simulink model "PID_miniHopper_4_Pitch_Roll_Yaw_Contour_4"  (R2022b)
settings: Solver=VariableStepAuto  StartTime=0.0  StopTime=10  RelTol=1e-3
values from neighbouring files (symbols this model uses):
  hopper_ode = struct()    [MiniHopperParameters.m]
undefined symbols (not defined in the file or in its folder): A_rpy, B_rpy, Gain_pitch_U, Gain_roll_U, Gain_yaw_U, kT, VxLoop, VyLoop, XIC_rpy, XLoop, YLoop
libraries: simulink_extras x16, slpidlib x10
(part 1 of 2)
settings Model: Creator=User  LastModifiedBy=User

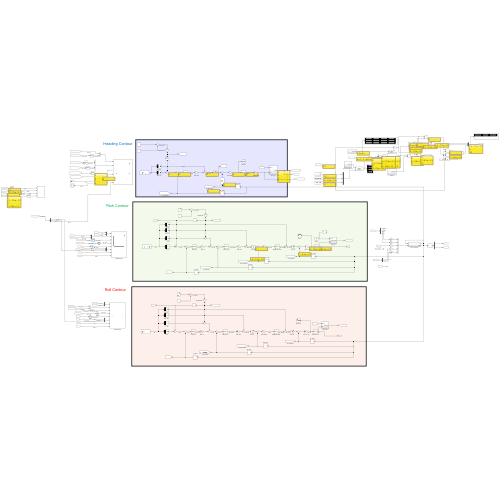
[thumbnail: Simulink's stored preview of the top-level diagram]
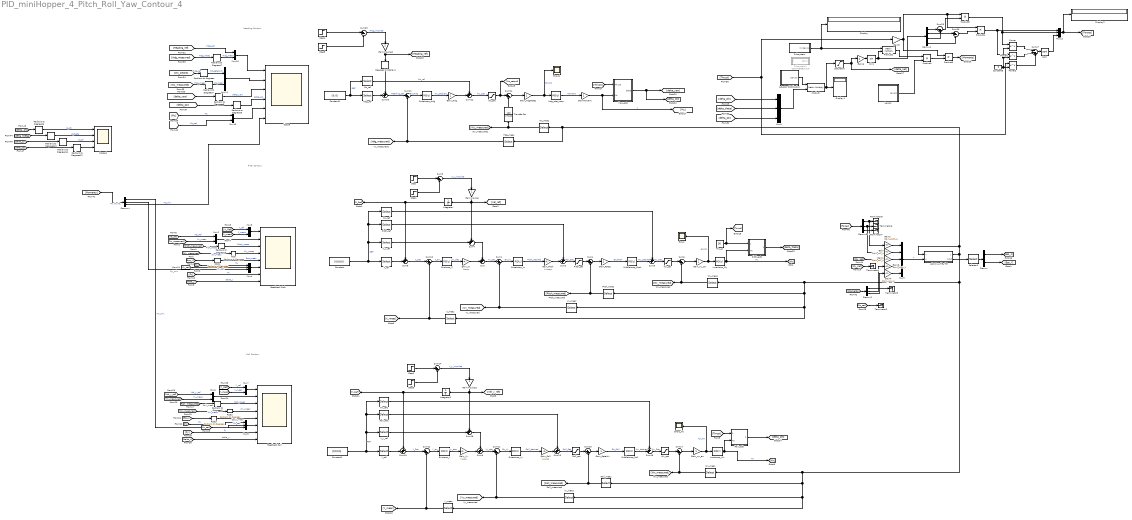
== system PID_miniHopper_4_Pitch_Roll_Yaw_Contour_4 ==
  note: Pitch Contour
  note: Roll Contour
  note: Heading Contour
  Actuator Distribution : Subsystem
  Constant : Constant  Value=[0;0;0;0]
  Constant1 : Constant  Value=[0;0;0;0]
  Constant2 : Constant  Value=[0; 0]
  Constant5 : Constant  Value=2
  Degrees to Radians : simulink_extras/Transformations/Degrees to Radians
  Demux : Demux  Outputs=2
  Demux1 : Demux
  Demux2 : Demux  Outputs=3
  Demux3 : Demux  Outputs=3
  Demux4 : Demux  Outputs=3
  Display : Display
  Display1 : Display
  Display2 : Display
  Errors : Scope
  Errors1 : Scope
  Errors_Wx : Scope
  ExoLoop_Y : slpidlib/PID Controller  Controller=PID  Form=Parallel  TimeDomain=Discrete-time  UseExternalTs=off  SampleTime=0.01  IntegratorMethod=Forward Euler  FilterMethod=Forward Euler  ControllerParametersSource=internal  P=0.1  I=0  UseKiTs=off  D=0  N=100  UseFilter=on  TunerSelectOption=Transfer Function Based (PID Tuner App)  InitialConditionSource=internal  InitialConditionForIntegrator=0  InitialConditionForFilter=0  DifferentiatorICPrevScaledInput=0  ExternalReset=none  TrackingMode=off  Kt=1  LimitOutput=off  SatLimitsSource=internal  UpperSaturationLimit=inf  LowerSaturationLimit=-inf  LinearizeAsGain=on  AntiWindupMode=none  Kb=1  LimitIntegrator=off  UpperIntegratorSaturationLimit=inf  LowerIntegratorSaturationLimit=-inf  POutMin=[]  POutMax=[]  IOutMin=[]  IOutMax=[]  DOutMin=[]  DOutMax=[]  NOutMin=[]  NOutMax=[]  SumOutMin=[]  SumOutMax=[]  SaturationOutMin=[]  SaturationOutMax=[]  PParamMin=[]  PParamMax=[]  IParamMin=[]  IParamMax=[]  DParamMin=[]  DParamMax=[]  NParamMin=[]  NParamMax=[]  KbParamMin=[]  KbParamMax=[]  KtParamMin=[]  KtParamMax=[]  KbOutMin=[]  KbOutMax=[]  KtOutMin=[]  KtOutMax=[]  IntegratorOutMin=[]  IntegratorOutMax=[]  FilterOutMin=[]  FilterOutMax=[]  SumI1OutMin=[]  SumI1OutMax=[]  SumI2OutMin=[]  SumI2OutMax=[]  SumI3OutMin=[]  SumI3OutMax=[]  SumI4OutMin=[]  SumI4OutMax=[]  SumDOutMin=[]  SumDOutMax=[]  DifferentiatorOutMin=[]  DifferentiatorOutMax=[]  FilterDiffOutCoefMin=[]  FilterDiffOutCoefMax=[]  ReciprocalOutMin=[]  ReciprocalOutMax=[]  SumDenOutMin=[]  SumDenOutMax=[]  SumNumOutMin=[]  SumNumOutMax=[]  DivideOutMin=[]  DivideOutMax=[]  UdiffTsProdOutMin=[]  UdiffTsProdOutMax=[]  NTsProdOutMin=[]  NTsProdOutMax=[]  UintegralTsProdOutMin=[]  UintegralTsProdOutMax=[]  UngainTsProdOutMin=[]  UngainTsProdOutMax=[]  ClampingZeroOutDataTypeStr=Inherit: Inherit via back propagation  ClampingZeroOutMin=[]  ClampingZeroOutMax=[]  FilterDenConstantOutDataTypeStr=Inherit: Inherit via back propagation  FilterDenConstantOutMin=[]  FilterDenConstantOutMax=[]  PCopyOutDataTypeStr=Inherit: Inherit via back propagation  PCopyOutMin=[]  PCopyOutMax=[]  NCopyOutDataTypeStr=Inherit: Inherit via back propagation  NCopyOutMin=[]  NCopyOutMax=[]  IntegratorContinuousStateAttributes=''  IntegratorStateMustResolveToSignalObject=off  IntegratorRTWStateStorageClass=Auto  FilterContinuousStateAttributes=''  FilterStateMustResolveToSignalObject=off  FilterRTWStateStorageClass=Auto  ParallelPVariant=InternalParameters  IdealPVariant=Disabled  IVariant=InternalParameters  DVariant=InternalParameters  IntegratorVariant=Discrete  SatVariant=Disabled  AWVariant=Passthrough  PCopyVariant=Disabled  TRVariant=Disabled  FdbkBlocksVariant=Forward  IdealPFdbkVariant=Disabled  SatFdbkVariant=Disabled  DerivativeFilterVariant=ForwardEulerFilter  NVariant=InternalParameters  NCopyVariant=Disabled  FilterICVariant=InternalICsFilter  IntegratorICVariant=InternalICs  ExternalResetVariant=Disabled  TRSumVariant=Passthrough  SumFdbkVariant=Disabled  SumVariant=Sum_PID  TsampFilterVariant=InternalTs  TsampNgainVariant=Passthrough  TsampIntegralVariant=Passthrough  ExternalSaturationOutDataTypeStr=Inherit: Same as second input
  ExoLoop_Z : slpidlib/PID Controller  Controller=PID  Form=Parallel  TimeDomain=Discrete-time  UseExternalTs=off  SampleTime=0.01  IntegratorMethod=Forward Euler  FilterMethod=Forward Euler  ControllerParametersSource=internal  P=0.1  I=0  UseKiTs=off  D=0  N=100  UseFilter=on  TunerSelectOption=Transfer Function Based (PID Tuner App)  InitialConditionSource=internal  InitialConditionForIntegrator=0  InitialConditionForFilter=0  DifferentiatorICPrevScaledInput=0  ExternalReset=none  TrackingMode=off  Kt=1  LimitOutput=off  SatLimitsSource=internal  UpperSaturationLimit=inf  LowerSaturationLimit=-inf  LinearizeAsGain=on  AntiWindupMode=none  Kb=1  LimitIntegrator=off  UpperIntegratorSaturationLimit=inf  LowerIntegratorSaturationLimit=-inf  POutMin=[]  POutMax=[]  IOutMin=[]  IOutMax=[]  DOutMin=[]  DOutMax=[]  NOutMin=[]  NOutMax=[]  SumOutMin=[]  SumOutMax=[]  SaturationOutMin=[]  SaturationOutMax=[]  PParamMin=[]  PParamMax=[]  IParamMin=[]  IParamMax=[]  DParamMin=[]  DParamMax=[]  NParamMin=[]  NParamMax=[]  KbParamMin=[]  KbParamMax=[]  KtParamMin=[]  KtParamMax=[]  KbOutMin=[]  KbOutMax=[]  KtOutMin=[]  KtOutMax=[]  IntegratorOutMin=[]  IntegratorOutMax=[]  FilterOutMin=[]  FilterOutMax=[]  SumI1OutMin=[]  SumI1OutMax=[]  SumI2OutMin=[]  SumI2OutMax=[]  SumI3OutMin=[]  SumI3OutMax=[]  SumI4OutMin=[]  SumI4OutMax=[]  SumDOutMin=[]  SumDOutMax=[]  DifferentiatorOutMin=[]  DifferentiatorOutMax=[]  FilterDiffOutCoefMin=[]  FilterDiffOutCoefMax=[]  ReciprocalOutMin=[]  ReciprocalOutMax=[]  SumDenOutMin=[]  SumDenOutMax=[]  SumNumOutMin=[]  SumNumOutMax=[]  DivideOutMin=[]  DivideOutMax=[]  UdiffTsProdOutMin=[]  UdiffTsProdOutMax=[]  NTsProdOutMin=[]  NTsProdOutMax=[]  UintegralTsProdOutMin=[]  UintegralTsProdOutMax=[]  UngainTsProdOutMin=[]  UngainTsProdOutMax=[]  ClampingZeroOutDataTypeStr=Inherit: Inherit via back propagation  ClampingZeroOutMin=[]  ClampingZeroOutMax=[]  FilterDenConstantOutDataTypeStr=Inherit: Inherit via back propagation  FilterDenConstantOutMin=[]  FilterDenConstantOutMax=[]  PCopyOutDataTypeStr=Inherit: Inherit via back propagation  PCopyOutMin=[]  PCopyOutMax=[]  NCopyOutDataTypeStr=Inherit: Inherit via back propagation  NCopyOutMin=[]  NCopyOutMax=[]  IntegratorContinuousStateAttributes=''  IntegratorStateMustResolveToSignalObject=off  IntegratorRTWStateStorageClass=Auto  FilterContinuousStateAttributes=''  FilterStateMustResolveToSignalObject=off  FilterRTWStateStorageClass=Auto  ParallelPVariant=InternalParameters  IdealPVariant=Disabled  IVariant=InternalParameters  DVariant=InternalParameters  IntegratorVariant=Discrete  SatVariant=Disabled  AWVariant=Passthrough  PCopyVariant=Disabled  TRVariant=Disabled  FdbkBlocksVariant=Forward  IdealPFdbkVariant=Disabled  SatFdbkVariant=Disabled  DerivativeFilterVariant=ForwardEulerFilter  NVariant=InternalParameters  NCopyVariant=Disabled  FilterICVariant=InternalICsFilter  IntegratorICVariant=InternalICs  ExternalResetVariant=Disabled  TRSumVariant=Passthrough  SumFdbkVariant=Disabled  SumVariant=Sum_PID  TsampFilterVariant=InternalTs  TsampNgainVariant=Passthrough  TsampIntegralVariant=Passthrough  ExternalSaturationOutDataTypeStr=Inherit: Same as second input
  Feedback Pitch : Scope  NumInputPorts=8
  Feedback Roll : Scope  NumInputPorts=8
  Gain : Gain  Gain=Gain_roll_U
  Gain1 : Gain  Gain=Gain_roll_U
  Gain2 : Gain  Gain=Gain_pitch_U
  Gain3 : Gain  Gain=Gain_pitch_U
  Gain4 : Gain  Gain=Gain_yaw_U
  Gain5 : Gain  Gain=kT *0.5
  Gain6 : Gain  Gain=2
  GainImpulse : Gain
  GainImpulse1 : Gain
  GainImpulse2 : Gain  Gain=2
  GainMoment : Gain
  Gain_Hdg : Gain
  Gain_HdgRates : Gain
  Gain_Pitch : Gain  Gain=VxLoop
  Gain_RateWx : Gain
  Gain_Rates : Gain
  Gain_Roll : Gain  Gain=VyLoop
  Gain_Vx : Gain  Gain=XLoop
  Gain_Vy : Gain  Gain=YLoop
  Gain_wx_err : Gain
  Gain_wy_err : Gain
  Hdg_meas : Selector  InputPortWidth=10  IndexOptions=Index vector (dialog)  Indices=[7]  OutputSizes=1
  Hdg_rate_Loop : slpidlib/PID Controller  Controller=PID  Form=Parallel  TimeDomain=Discrete-time  UseExternalTs=off  SampleTime=0.001  IntegratorMethod=Forward Euler  FilterMethod=Forward Euler  ControllerParametersSource=internal  P=0.8  I=0  UseKiTs=off  D=0  N=100  UseFilter=on  TunerSelectOption=Transfer Function Based (PID Tuner App)  InitialConditionSource=internal  InitialConditionForIntegrator=0  InitialConditionForFilter=0  DifferentiatorICPrevScaledInput=0  ExternalReset=none  TrackingMode=off  Kt=1  LimitOutput=off  SatLimitsSource=internal  UpperSaturationLimit=inf  LowerSaturationLimit=-inf  LinearizeAsGain=on  AntiWindupMode=none  Kb=1  LimitIntegrator=off  UpperIntegratorSaturationLimit=inf  LowerIntegratorSaturationLimit=-inf  POutMin=[]  POutMax=[]  IOutMin=[]  IOutMax=[]  DOutMin=[]  DOutMax=[]  NOutMin=[]  NOutMax=[]  SumOutMin=[]  SumOutMax=[]  SaturationOutMin=[]  SaturationOutMax=[]  PParamMin=[]  PParamMax=[]  IParamMin=[]  IParamMax=[]  DParamMin=[]  DParamMax=[]  NParamMin=[]  NParamMax=[]  KbParamMin=[]  KbParamMax=[]  KtParamMin=[]  KtParamMax=[]  KbOutMin=[]  KbOutMax=[]  KtOutMin=[]  KtOutMax=[]  IntegratorOutMin=[]  IntegratorOutMax=[]  FilterOutMin=[]  FilterOutMax=[]  SumI1OutMin=[]  SumI1OutMax=[]  SumI2OutMin=[]  SumI2OutMax=[]  SumI3OutMin=[]  SumI3OutMax=[]  SumI4OutMin=[]  SumI4OutMax=[]  SumDOutMin=[]  SumDOutMax=[]  DifferentiatorOutMin=[]  DifferentiatorOutMax=[]  FilterDiffOutCoefMin=[]  FilterDiffOutCoefMax=[]  ReciprocalOutMin=[]  ReciprocalOutMax=[]  SumDenOutMin=[]  SumDenOutMax=[]  SumNumOutMin=[]  SumNumOutMax=[]  DivideOutMin=[]  DivideOutMax=[]  UdiffTsProdOutMin=[]  UdiffTsProdOutMax=[]  NTsProdOutMin=[]  NTsProdOutMax=[]  UintegralTsProdOutMin=[]  UintegralTsProdOutMax=[]  UngainTsProdOutMin=[]  UngainTsProdOutMax=[]  ClampingZeroOutDataTypeStr=Inherit: Inherit via back propagation  ClampingZeroOutMin=[]  ClampingZeroOutMax=[]  FilterDenConstantOutDataTypeStr=Inherit: Inherit via back propagation  FilterDenConstantOutMin=[]  FilterDenConstantOutMax=[]  PCopyOutDataTypeStr=Inherit: Inherit via back propagation  PCopyOutMin=[]  PCopyOutMax=[]  NCopyOutDataTypeStr=Inherit: Inherit via back propagation  NCopyOutMin=[]  NCopyOutMax=[]  IntegratorContinuousStateAttributes=''  IntegratorStateMustResolveToSignalObject=off  IntegratorRTWStateStorageClass=Auto  FilterContinuousStateAttributes=''  FilterStateMustResolveToSignalObject=off  FilterRTWStateStorageClass=Auto  ParallelPVariant=InternalParameters  IdealPVariant=Disabled  IVariant=InternalParameters  DVariant=InternalParameters  IntegratorVariant=Discrete  SatVariant=Disabled  AWVariant=Passthrough  PCopyVariant=Disabled  TRVariant=Disabled  FdbkBlocksVariant=Forward  IdealPFdbkVariant=Disabled  SatFdbkVariant=Disabled  DerivativeFilterVariant=ForwardEulerFilter  NVariant=InternalParameters  NCopyVariant=Disabled  FilterICVariant=InternalICsFilter  IntegratorICVariant=InternalICs  ExternalResetVariant=Disabled  TRSumVariant=Passthrough  SumFdbkVariant=Disabled  SumVariant=Sum_PID  TsampFilterVariant=InternalTs  TsampNgainVariant=Passthrough  TsampIntegralVariant=Passthrough  ExternalSaturationOutDataTypeStr=Inherit: Same as second input
  Hdg_ref : Selector  InputPortWidth=2  IndexOptions=Index vector (dialog)  Indices=[1]  OutputSizes=1
  InnerLoop_Wx : slpidlib/PID Controller  Controller=PID  Form=Parallel  TimeDomain=Discrete-time  UseExternalTs=off  SampleTime=0.001  IntegratorMethod=Forward Euler  FilterMethod=Forward Euler  ControllerParametersSource=internal  P=10  I=0  UseKiTs=off  D=0.015  N=100  UseFilter=on  TunerSelectOption=Transfer Function Based (PID Tuner App)  InitialConditionSource=internal  InitialConditionForIntegrator=0  InitialConditionForFilter=0  DifferentiatorICPrevScaledInput=0  ExternalReset=none  TrackingMode=off  Kt=1  LimitOutput=off  SatLimitsSource=internal  UpperSaturationLimit=inf  LowerSaturationLimit=-inf  LinearizeAsGain=on  AntiWindupMode=none  Kb=1  LimitIntegrator=off  UpperIntegratorSaturationLimit=inf  LowerIntegratorSaturationLimit=-inf  POutMin=[]  POutMax=[]  IOutMin=[]  IOutMax=[]  DOutMin=[]  DOutMax=[]  NOutMin=[]  NOutMax=[]  SumOutMin=[]  SumOutMax=[]  SaturationOutMin=[]  SaturationOutMax=[]  PParamMin=[]  PParamMax=[]  IParamMin=[]  IParamMax=[]  DParamMin=[]  DParamMax=[]  NParamMin=[]  NParamMax=[]  KbParamMin=[]  KbParamMax=[]  KtParamMin=[]  KtParamMax=[]  KbOutMin=[]  KbOutMax=[]  KtOutMin=[]  KtOutMax=[]  IntegratorOutMin=[]  IntegratorOutMax=[]  FilterOutMin=[]  FilterOutMax=[]  SumI1OutMin=[]  SumI1OutMax=[]  SumI2OutMin=[]  SumI2OutMax=[]  SumI3OutMin=[]  SumI3OutMax=[]  SumI4OutMin=[]  SumI4OutMax=[]  SumDOutMin=[]  SumDOutMax=[]  DifferentiatorOutMin=[]  DifferentiatorOutMax=[]  FilterDiffOutCoefMin=[]  FilterDiffOutCoefMax=[]  ReciprocalOutMin=[]  ReciprocalOutMax=[]  SumDenOutMin=[]  SumDenOutMax=[]  SumNumOutMin=[]  SumNumOutMax=[]  DivideOutMin=[]  DivideOutMax=[]  UdiffTsProdOutMin=[]  UdiffTsProdOutMax=[]  NTsProdOutMin=[]  NTsProdOutMax=[]  UintegralTsProdOutMin=[]  UintegralTsProdOutMax=[]  UngainTsProdOutMin=[]  UngainTsProdOutMax=[]  ClampingZeroOutDataTypeStr=Inherit: Inherit via back propagation  ClampingZeroOutMin=[]  ClampingZeroOutMax=[]  FilterDenConstantOutDataTypeStr=Inherit: Inherit via back propagation  FilterDenConstantOutMin=[]  FilterDenConstantOutMax=[]  PCopyOutDataTypeStr=Inherit: Inherit via back propagation  PCopyOutMin=[]  PCopyOutMax=[]  NCopyOutDataTypeStr=Inherit: Inherit via back propagation  NCopyOutMin=[]  NCopyOutMax=[]  IntegratorContinuousStateAttributes=''  IntegratorStateMustResolveToSignalObject=off  IntegratorRTWStateStorageClass=Auto  FilterContinuousStateAttributes=''  FilterStateMustResolveToSignalObject=off  FilterRTWStateStorageClass=Auto  ParallelPVariant=InternalParameters  IdealPVariant=Disabled  IVariant=InternalParameters  DVariant=InternalParameters  IntegratorVariant=Discrete  SatVariant=Disabled  AWVariant=Passthrough  PCopyVariant=Disabled  TRVariant=Disabled  FdbkBlocksVariant=Forward  IdealPFdbkVariant=Disabled  SatFdbkVariant=Disabled  DerivativeFilterVariant=ForwardEulerFilter  NVariant=InternalParameters  NCopyVariant=Disabled  FilterICVariant=InternalICsFilter  IntegratorICVariant=InternalICs  ExternalResetVariant=Disabled  TRSumVariant=Passthrough  SumFdbkVariant=Disabled  SumVariant=Sum_PID  TsampFilterVariant=InternalTs  TsampNgainVariant=Passthrough  TsampIntegralVariant=Passthrough  ExternalSaturationOutDataTypeStr=Inherit: Same as second input
  InnerLoop_Wy : slpidlib/PID Controller  Controller=PID  Form=Parallel  TimeDomain=Discrete-time  UseExternalTs=off  SampleTime=0.001  IntegratorMethod=Forward Euler  FilterMethod=Forward Euler  ControllerParametersSource=internal  P=10  I=0  UseKiTs=off  D=0.015  N=100  UseFilter=on  TunerSelectOption=Transfer Function Based (PID Tuner App)  InitialConditionSource=internal  InitialConditionForIntegrator=0  InitialConditionForFilter=0  DifferentiatorICPrevScaledInput=0  ExternalReset=none  TrackingMode=off  Kt=1  LimitOutput=off  SatLimitsSource=internal  UpperSaturationLimit=inf  LowerSaturationLimit=-inf  LinearizeAsGain=on  AntiWindupMode=none  Kb=1  LimitIntegrator=off  UpperIntegratorSaturationLimit=inf  LowerIntegratorSaturationLimit=-inf  POutMin=[]  POutMax=[]  IOutMin=[]  IOutMax=[]  DOutMin=[]  DOutMax=[]  NOutMin=[]  NOutMax=[]  SumOutMin=[]  SumOutMax=[]  SaturationOutMin=[]  SaturationOutMax=[]  PParamMin=[]  PParamMax=[]  IParamMin=[]  IParamMax=[]  DParamMin=[]  DParamMax=[]  NParamMin=[]  NParamMax=[]  KbParamMin=[]  KbParamMax=[]  KtParamMin=[]  KtParamMax=[]  KbOutMin=[]  KbOutMax=[]  KtOutMin=[]  KtOutMax=[]  IntegratorOutMin=[]  IntegratorOutMax=[]  FilterOutMin=[]  FilterOutMax=[]  SumI1OutMin=[]  SumI1OutMax=[]  SumI2OutMin=[]  SumI2OutMax=[]  SumI3OutMin=[]  SumI3OutMax=[]  SumI4OutMin=[]  SumI4OutMax=[]  SumDOutMin=[]  SumDOutMax=[]  DifferentiatorOutMin=[]  DifferentiatorOutMax=[]  FilterDiffOutCoefMin=[]  FilterDiffOutCoefMax=[]  ReciprocalOutMin=[]  ReciprocalOutMax=[]  SumDenOutMin=[]  SumDenOutMax=[]  SumNumOutMin=[]  SumNumOutMax=[]  DivideOutMin=[]  DivideOutMax=[]  UdiffTsProdOutMin=[]  UdiffTsProdOutMax=[]  NTsProdOutMin=[]  NTsProdOutMax=[]  UintegralTsProdOutMin=[]  UintegralTsProdOutMax=[]  UngainTsProdOutMin=[]  UngainTsProdOutMax=[]  ClampingZeroOutDataTypeStr=Inherit: Inherit via back propagation  ClampingZeroOutMin=[]  ClampingZeroOutMax=[]  FilterDenConstantOutDataTypeStr=Inherit: Inherit via back propagation  FilterDenConstantOutMin=[]  FilterDenConstantOutMax=[]  PCopyOutDataTypeStr=Inherit: Inherit via back propagation  PCopyOutMin=[]  PCopyOutMax=[]  NCopyOutDataTypeStr=Inherit: Inherit via back propagation  NCopyOutMin=[]  NCopyOutMax=[]  IntegratorContinuousStateAttributes=''  IntegratorStateMustResolveToSignalObject=off  IntegratorRTWStateStorageClass=Auto  FilterContinuousStateAttributes=''  FilterStateMustResolveToSignalObject=off  FilterRTWStateStorageClass=Auto  ParallelPVariant=InternalParameters  IdealPVariant=Disabled  IVariant=InternalParameters  DVariant=InternalParameters  IntegratorVariant=Discrete  SatVariant=Disabled  AWVariant=Passthrough  PCopyVariant=Disabled  TRVariant=Disabled  FdbkBlocksVariant=Forward  IdealPFdbkVariant=Disabled  SatFdbkVariant=Disabled  DerivativeFilterVariant=ForwardEulerFilter  NVariant=InternalParameters  NCopyVariant=Disabled  FilterICVariant=InternalICsFilter  IntegratorICVariant=InternalICs  ExternalResetVariant=Disabled  TRSumVariant=Passthrough  SumFdbkVariant=Disabled  SumVariant=Sum_PID  TsampFilterVariant=InternalTs  TsampNgainVariant=Passthrough  TsampIntegralVariant=Passthrough  ExternalSaturationOutDataTypeStr=Inherit: Same as second input
  Integrator : Integrator
  Integrator1 : Integrator
  Levers : Subsystem
  MiddleLoop_Pitch : slpidlib/PID Controller  Controller=PID  Form=Parallel  TimeDomain=Discrete-time  UseExternalTs=off  SampleTime=0.001  IntegratorMethod=Forward Euler  FilterMethod=Forward Euler  ControllerParametersSource=internal  P=10  I=0.0012  UseKiTs=off  D=0.5  N=100  UseFilter=on  TunerSelectOption=Transfer Function Based (PID Tuner App)  InitialConditionSource=internal  InitialConditionForIntegrator=0  InitialConditionForFilter=0  DifferentiatorICPrevScaledInput=0  ExternalReset=none  TrackingMode=off  Kt=1  LimitOutput=off  SatLimitsSource=internal  UpperSaturationLimit=inf  LowerSaturationLimit=-inf  LinearizeAsGain=on  AntiWindupMode=none  Kb=1  LimitIntegrator=off  UpperIntegratorSaturationLimit=inf  LowerIntegratorSaturationLimit=-inf  POutMin=[]  POutMax=[]  IOutMin=[]  IOutMax=[]  DOutMin=[]  DOutMax=[]  NOutMin=[]  NOutMax=[]  SumOutMin=[]  SumOutMax=[]  SaturationOutMin=[]  SaturationOutMax=[]  PParamMin=[]  PParamMax=[]  IParamMin=[]  IParamMax=[]  DParamMin=[]  DParamMax=[]  NParamMin=[]  NParamMax=[]  KbParamMin=[]  KbParamMax=[]  KtParamMin=[]  KtParamMax=[]  KbOutMin=[]  KbOutMax=[]  KtOutMin=[]  KtOutMax=[]  IntegratorOutMin=[]  IntegratorOutMax=[]  FilterOutMin=[]  FilterOutMax=[]  SumI1OutMin=[]  SumI1OutMax=[]  SumI2OutMin=[]  SumI2OutMax=[]  SumI3OutMin=[]  SumI3OutMax=[]  SumI4OutMin=[]  SumI4OutMax=[]  SumDOutMin=[]  SumDOutMax=[]  DifferentiatorOutMin=[]  DifferentiatorOutMax=[]  FilterDiffOutCoefMin=[]  FilterDiffOutCoefMax=[]  ReciprocalOutMin=[]  ReciprocalOutMax=[]  SumDenOutMin=[]  SumDenOutMax=[]  SumNumOutMin=[]  SumNumOutMax=[]  DivideOutMin=[]  DivideOutMax=[]  UdiffTsProdOutMin=[]  UdiffTsProdOutMax=[]  NTsProdOutMin=[]  NTsProdOutMax=[]  UintegralTsProdOutMin=[]  UintegralTsProdOutMax=[]  UngainTsProdOutMin=[]  UngainTsProdOutMax=[]  ClampingZeroOutDataTypeStr=Inherit: Inherit via back propagation  ClampingZeroOutMin=[]  ClampingZeroOutMax=[]  FilterDenConstantOutDataTypeStr=Inherit: Inherit via back propagation  FilterDenConstantOutMin=[]  FilterDenConstantOutMax=[]  PCopyOutDataTypeStr=Inherit: Inherit via back propagation  PCopyOutMin=[]  PCopyOutMax=[]  NCopyOutDataTypeStr=Inherit: Inherit via back propagation  NCopyOutMin=[]  NCopyOutMax=[]  IntegratorContinuousStateAttributes=''  IntegratorStateMustResolveToSignalObject=off  IntegratorRTWStateStorageClass=Auto  FilterContinuousStateAttributes=''  FilterStateMustResolveToSignalObject=off  FilterRTWStateStorageClass=Auto  ParallelPVariant=InternalParameters  IdealPVariant=Disabled  IVariant=InternalParameters  DVariant=InternalParameters  IntegratorVariant=Discrete  SatVariant=Disabled  AWVariant=Passthrough  PCopyVariant=Disabled  TRVariant=Disabled  FdbkBlocksVariant=Forward  IdealPFdbkVariant=Disabled  SatFdbkVariant=Disabled  DerivativeFilterVariant=ForwardEulerFilter  NVariant=InternalParameters  NCopyVariant=Disabled  FilterICVariant=InternalICsFilter  IntegratorICVariant=InternalICs  ExternalResetVariant=Disabled  TRSumVariant=Passthrough  SumFdbkVariant=Disabled  SumVariant=Sum_PID  TsampFilterVariant=InternalTs  TsampNgainVariant=Passthrough  TsampIntegralVariant=Passthrough  ExternalSaturationOutDataTypeStr=Inherit: Same as second input
  MiddleLoop_Roll : slpidlib/PID Controller  Controller=PID  Form=Parallel  TimeDomain=Discrete-time  UseExternalTs=off  SampleTime=0.001  IntegratorMethod=Forward Euler  FilterMethod=Forward Euler  ControllerParametersSource=internal  P=10  I=0.0012  UseKiTs=off  D=0.5  N=100  UseFilter=on  TunerSelectOption=Transfer Function Based (PID Tuner App)  InitialConditionSource=internal  InitialConditionForIntegrator=0  InitialConditionForFilter=0  DifferentiatorICPrevScaledInput=0  ExternalReset=none  TrackingMode=off  Kt=1  LimitOutput=off  SatLimitsSource=internal  UpperSaturationLimit=inf  LowerSaturationLimit=-inf  LinearizeAsGain=on  AntiWindupMode=none  Kb=1  LimitIntegrator=off  UpperIntegratorSaturationLimit=inf  LowerIntegratorSaturationLimit=-inf  POutMin=[]  POutMax=[]  IOutMin=[]  IOutMax=[]  DOutMin=[]  DOutMax=[]  NOutMin=[]  NOutMax=[]  SumOutMin=[]  SumOutMax=[]  SaturationOutMin=[]  SaturationOutMax=[]  PParamMin=[]  PParamMax=[]  IParamMin=[]  IParamMax=[]  DParamMin=[]  DParamMax=[]  NParamMin=[]  NParamMax=[]  KbParamMin=[]  KbParamMax=[]  KtParamMin=[]  KtParamMax=[]  KbOutMin=[]  KbOutMax=[]  KtOutMin=[]  KtOutMax=[]  IntegratorOutMin=[]  IntegratorOutMax=[]  FilterOutMin=[]  FilterOutMax=[]  SumI1OutMin=[]  SumI1OutMax=[]  SumI2OutMin=[]  SumI2OutMax=[]  SumI3OutMin=[]  SumI3OutMax=[]  SumI4OutMin=[]  SumI4OutMax=[]  SumDOutMin=[]  SumDOutMax=[]  DifferentiatorOutMin=[]  DifferentiatorOutMax=[]  FilterDiffOutCoefMin=[]  FilterDiffOutCoefMax=[]  ReciprocalOutMin=[]  ReciprocalOutMax=[]  SumDenOutMin=[]  SumDenOutMax=[]  SumNumOutMin=[]  SumNumOutMax=[]  DivideOutMin=[]  DivideOutMax=[]  UdiffTsProdOutMin=[]  UdiffTsProdOutMax=[]  NTsProdOutMin=[]  NTsProdOutMax=[]  UintegralTsProdOutMin=[]  UintegralTsProdOutMax=[]  UngainTsProdOutMin=[]  UngainTsProdOutMax=[]  ClampingZeroOutDataTypeStr=Inherit: Inherit via back propagation  ClampingZeroOutMin=[]  ClampingZeroOutMax=[]  FilterDenConstantOutDataTypeStr=Inherit: Inherit via back propagation  FilterDenConstantOutMin=[]  FilterDenConstantOutMax=[]  PCopyOutDataTypeStr=Inherit: Inherit via back propagation  PCopyOutMin=[]  PCopyOutMax=[]  NCopyOutDataTypeStr=Inherit: Inherit via back propagation  NCopyOutMin=[]  NCopyOutMax=[]  IntegratorContinuousStateAttributes=''  IntegratorStateMustResolveToSignalObject=off  IntegratorRTWStateStorageClass=Auto  FilterContinuousStateAttributes=''  FilterStateMustResolveToSignalObject=off  FilterRTWStateStorageClass=Auto  ParallelPVariant=InternalParameters  IdealPVariant=Disabled  IVariant=InternalParameters  DVariant=InternalParameters  IntegratorVariant=Discrete  SatVariant=Disabled  AWVariant=Passthrough  PCopyVariant=Disabled  TRVariant=Disabled  FdbkBlocksVariant=Forward  IdealPFdbkVariant=Disabled  SatFdbkVariant=Disabled  DerivativeFilterVariant=ForwardEulerFilter  NVariant=InternalParameters  NCopyVariant=Disabled  FilterICVariant=InternalICsFilter  IntegratorICVariant=InternalICs  ExternalResetVariant=Disabled  TRSumVariant=Passthrough  SumFdbkVariant=Disabled  SumVariant=Sum_PID  TsampFilterVariant=InternalTs  TsampNgainVariant=Passthrough  TsampIntegralVariant=Passthrough  ExternalSaturationOutDataTypeStr=Inherit: Same as second input
  Mux{2..3,6..7,10..11,13} (7 alike) : Mux  Inputs=2
  Mux{4,8..9,12} (4 alike) : Mux  Inputs=3
  Mux5 : Mux  Inputs=5
  OuterLoop_Hdg : slpidlib/PID Controller  Controller=PID  Form=Parallel  TimeDomain=Discrete-time  UseExternalTs=off  SampleTime=0.01  IntegratorMethod=Forward Euler  FilterMethod=Forward Euler  ControllerParametersSource=internal  P=10  I=0  UseKiTs=off  D=0  N=100  UseFilter=on  TunerSelectOption=Transfer Function Based (PID Tuner App)  InitialConditionSource=internal  InitialConditionForIntegrator=0  InitialConditionForFilter=0  DifferentiatorICPrevScaledInput=0  ExternalReset=none  TrackingMode=off  Kt=1  LimitOutput=off  SatLimitsSource=internal  UpperSaturationLimit=inf  LowerSaturationLimit=-inf  LinearizeAsGain=on  AntiWindupMode=none  Kb=1  LimitIntegrator=off  UpperIntegratorSaturationLimit=inf  LowerIntegratorSaturationLimit=-inf  POutMin=[]  POutMax=[]  IOutMin=[]  IOutMax=[]  DOutMin=[]  DOutMax=[]  NOutMin=[]  NOutMax=[]  SumOutMin=[]  SumOutMax=[]  SaturationOutMin=[]  SaturationOutMax=[]  PParamMin=[]  PParamMax=[]  IParamMin=[]  IParamMax=[]  DParamMin=[]  DParamMax=[]  NParamMin=[]  NParamMax=[]  KbParamMin=[]  KbParamMax=[]  KtParamMin=[]  KtParamMax=[]  KbOutMin=[]  KbOutMax=[]  KtOutMin=[]  KtOutMax=[]  IntegratorOutMin=[]  IntegratorOutMax=[]  FilterOutMin=[]  FilterOutMax=[]  SumI1OutMin=[]  SumI1OutMax=[]  SumI2OutMin=[]  SumI2OutMax=[]  SumI3OutMin=[]  SumI3OutMax=[]  SumI4OutMin=[]  SumI4OutMax=[]  SumDOutMin=[]  SumDOutMax=[]  DifferentiatorOutMin=[]  DifferentiatorOutMax=[]  FilterDiffOutCoefMin=[]  FilterDiffOutCoefMax=[]  ReciprocalOutMin=[]  ReciprocalOutMax=[]  SumDenOutMin=[]  SumDenOutMax=[]  SumNumOutMin=[]  SumNumOutMax=[]  DivideOutMin=[]  DivideOutMax=[]  UdiffTsProdOutMin=[]  UdiffTsProdOutMax=[]  NTsProdOutMin=[]  NTsProdOutMax=[]  UintegralTsProdOutMin=[]  UintegralTsProdOutMax=[]  UngainTsProdOutMin=[]  UngainTsProdOutMax=[]  ClampingZeroOutDataTypeStr=Inherit: Inherit via back propagation  ClampingZeroOutMin=[]  ClampingZeroOutMax=[]  FilterDenConstantOutDataTypeStr=Inherit: Inherit via back propagation  FilterDenConstantOutMin=[]  FilterDenConstantOutMax=[]  PCopyOutDataTypeStr=Inherit: Inherit via back propagation  PCopyOutMin=[]  PCopyOutMax=[]  NCopyOutDataTypeStr=Inherit: Inherit via back propagation  NCopyOutMin=[]  NCopyOutMax=[]  IntegratorContinuousStateAttributes=''  IntegratorStateMustResolveToSignalObject=off  IntegratorRTWStateStorageClass=Auto  FilterContinuousStateAttributes=''  FilterStateMustResolveToSignalObject=off  FilterRTWStateStorageClass=Auto  ParallelPVariant=InternalParameters  IdealPVariant=Disabled  IVariant=InternalParameters  DVariant=InternalParameters  IntegratorVariant=Discrete  SatVariant=Disabled  AWVariant=Passthrough  PCopyVariant=Disabled  TRVariant=Disabled  FdbkBlocksVariant=Forward  IdealPFdbkVariant=Disabled  SatFdbkVariant=Disabled  DerivativeFilterVariant=ForwardEulerFilter  NVariant=InternalParameters  NCopyVariant=Disabled  FilterICVariant=InternalICsFilter  IntegratorICVariant=InternalICs  ExternalResetVariant=Disabled  TRSumVariant=Passthrough  SumFdbkVariant=Disabled  SumVariant=Sum_PID  TsampFilterVariant=InternalTs  TsampNgainVariant=Passthrough  TsampIntegralVariant=Passthrough  ExternalSaturationOutDataTypeStr=Inherit: Same as second input
  OuterLoop_Vx : slpidlib/PID Controller  Controller=PID  Form=Parallel  TimeDomain=Discrete-time  UseExternalTs=off  SampleTime=0.01  IntegratorMethod=Forward Euler  FilterMethod=Forward Euler  ControllerParametersSource=internal  P=0.5  I=0  UseKiTs=off  D=0  N=100  UseFilter=on  TunerSelectOption=Transfer Function Based (PID Tuner App)  ZeroCross=off  InitialConditionSource=internal  InitialConditionForIntegrator=0  InitialConditionForFilter=0  DifferentiatorICPrevScaledInput=0  ExternalReset=none  TrackingMode=off  Kt=1  LimitOutput=off  SatLimitsSource=internal  UpperSaturationLimit=inf  LowerSaturationLimit=-inf  LinearizeAsGain=on  AntiWindupMode=none  Kb=1  LimitIntegrator=off  UpperIntegratorSaturationLimit=inf  LowerIntegratorSaturationLimit=-inf  POutMin=[]  POutMax=[]  IOutMin=[]  IOutMax=[]  DOutMin=[]  DOutMax=[]  NOutMin=[]  NOutMax=[]  SumOutMin=[]  SumOutMax=[]  SaturationOutMin=[]  SaturationOutMax=[]  PParamMin=[]  PParamMax=[]  IParamMin=[]  IParamMax=[]  DParamMin=[]  DParamMax=[]  NParamMin=[]  NParamMax=[]  KbParamMin=[]  KbParamMax=[]  KtParamMin=[]  KtParamMax=[]  KbOutMin=[]  KbOutMax=[]  KtOutMin=[]  KtOutMax=[]  IntegratorOutMin=[]  IntegratorOutMax=[]  FilterOutMin=[]  FilterOutMax=[]  SumI1OutMin=[]  SumI1OutMax=[]  SumI2OutMin=[]  SumI2OutMax=[]  SumI3OutMin=[]  SumI3OutMax=[]  SumI4OutMin=[]  SumI4OutMax=[]  SumDOutMin=[]  SumDOutMax=[]  DifferentiatorOutMin=[]  DifferentiatorOutMax=[]  FilterDiffOutCoefMin=[]  FilterDiffOutCoefMax=[]  ReciprocalOutMin=[]  ReciprocalOutMax=[]  SumDenOutMin=[]  SumDenOutMax=[]  SumNumOutMin=[]  SumNumOutMax=[]  DivideOutMin=[]  DivideOutMax=[]  UdiffTsProdOutMin=[]  UdiffTsProdOutMax=[]  NTsProdOutMin=[]  NTsProdOutMax=[]  UintegralTsProdOutMin=[]  UintegralTsProdOutMax=[]  UngainTsProdOutMin=[]  UngainTsProdOutMax=[]  ClampingZeroOutDataTypeStr=Inherit: Inherit via back propagation  ClampingZeroOutMin=[]  ClampingZeroOutMax=[]  FilterDenConstantOutDataTypeStr=Inherit: Inherit via back propagation  FilterDenConstantOutMin=[]  FilterDenConstantOutMax=[]  PCopyOutDataTypeStr=Inherit: Inherit via back propagation  PCopyOutMin=[]  PCopyOutMax=[]  NCopyOutDataTypeStr=Inherit: Inherit via back propagation  NCopyOutMin=[]  NCopyOutMax=[]  IntegratorContinuousStateAttributes=''  IntegratorStateMustResolveToSignalObject=off  IntegratorRTWStateStorageClass=Auto  FilterContinuousStateAttributes=''  FilterStateMustResolveToSignalObject=off  FilterRTWStateStorageClass=Auto  ParallelPVariant=InternalParameters  IdealPVariant=Disabled  IVariant=InternalParameters  DVariant=InternalParameters  IntegratorVariant=Discrete  SatVariant=Disabled  AWVariant=Passthrough  PCopyVariant=Disabled  TRVariant=Disabled  FdbkBlocksVariant=Forward  IdealPFdbkVariant=Disabled  SatFdbkVariant=Disabled  DerivativeFilterVariant=ForwardEulerFilter  NVariant=InternalParameters  NCopyVariant=Disabled  FilterICVariant=InternalICsFilter  IntegratorICVariant=InternalICs  ExternalResetVariant=Disabled  TRSumVariant=Passthrough  SumFdbkVariant=Disabled  SumVariant=Sum_PID  TsampFilterVariant=InternalTs  TsampNgainVariant=Passthrough  TsampIntegralVariant=Passthrough  ExternalSaturationOutDataTypeStr=Inherit: Same as second input
  OuterLoop_Vy : slpidlib/PID Controller  Controller=PID  Form=Parallel  TimeDomain=Discrete-time  UseExternalTs=off  SampleTime=0.01  IntegratorMethod=Forward Euler  FilterMethod=Forward Euler  ControllerParametersSource=internal  P=0.5  I=0  UseKiTs=off  D=0  N=100  UseFilter=on  TunerSelectOption=Transfer Function Based (PID Tuner App)  ZeroCross=off  InitialConditionSource=internal  InitialConditionForIntegrator=0  InitialConditionForFilter=0  DifferentiatorICPrevScaledInput=0  ExternalReset=none  TrackingMode=off  Kt=1  LimitOutput=off  SatLimitsSource=internal  UpperSaturationLimit=inf  LowerSaturationLimit=-inf  LinearizeAsGain=on  AntiWindupMode=none  Kb=1  LimitIntegrator=off  UpperIntegratorSaturationLimit=inf  LowerIntegratorSaturationLimit=-inf  POutMin=[]  POutMax=[]  IOutMin=[]  IOutMax=[]  DOutMin=[]  DOutMax=[]  NOutMin=[]  NOutMax=[]  SumOutMin=[]  SumOutMax=[]  SaturationOutMin=[]  SaturationOutMax=[]  PParamMin=[]  PParamMax=[]  IParamMin=[]  IParamMax=[]  DParamMin=[]  DParamMax=[]  NParamMin=[]  NParamMax=[]  KbParamMin=[]  KbParamMax=[]  KtParamMin=[]  KtParamMax=[]  KbOutMin=[]  KbOutMax=[]  KtOutMin=[]  KtOutMax=[]  IntegratorOutMin=[]  IntegratorOutMax=[]  FilterOutMin=[]  FilterOutMax=[]  SumI1OutMin=[]  SumI1OutMax=[]  SumI2OutMin=[]  SumI2OutMax=[]  SumI3OutMin=[]  SumI3OutMax=[]  SumI4OutMin=[]  SumI4OutMax=[]  SumDOutMin=[]  SumDOutMax=[]  DifferentiatorOutMin=[]  DifferentiatorOutMax=[]  FilterDiffOutCoefMin=[]  FilterDiffOutCoefMax=[]  ReciprocalOutMin=[]  ReciprocalOutMax=[]  SumDenOutMin=[]  SumDenOutMax=[]  SumNumOutMin=[]  SumNumOutMax=[]  DivideOutMin=[]  DivideOutMax=[]  UdiffTsProdOutMin=[]  UdiffTsProdOutMax=[]  NTsProdOutMin=[]  NTsProdOutMax=[]  UintegralTsProdOutMin=[]  UintegralTsProdOutMax=[]  UngainTsProdOutMin=[]  UngainTsProdOutMax=[]  ClampingZeroOutDataTypeStr=Inherit: Inherit via back propagation  ClampingZeroOutMin=[]  ClampingZeroOutMax=[]  FilterDenConstantOutDataTypeStr=Inherit: Inherit via back propagation  FilterDenConstantOutMin=[]  FilterDenConstantOutMax=[]  PCopyOutDataTypeStr=Inherit: Inherit via back propagation  PCopyOutMin=[]  PCopyOutMax=[]  NCopyOutDataTypeStr=Inherit: Inherit via back propagation  NCopyOutMin=[]  NCopyOutMax=[]  IntegratorContinuousStateAttributes=''  IntegratorStateMustResolveToSignalObject=off  IntegratorRTWStateStorageClass=Auto  FilterContinuousStateAttributes=''  FilterStateMustResolveToSignalObject=off  FilterRTWStateStorageClass=Auto  ParallelPVariant=InternalParameters  IdealPVariant=Disabled  IVariant=InternalParameters  DVariant=InternalParameters  IntegratorVariant=Discrete  SatVariant=Disabled  AWVariant=Passthrough  PCopyVariant=Disabled  TRVariant=Disabled  FdbkBlocksVariant=Forward  IdealPFdbkVariant=Disabled  SatFdbkVariant=Disabled  DerivativeFilterVariant=ForwardEulerFilter  NVariant=InternalParameters  NCopyVariant=Disabled  FilterICVariant=InternalICsFilter  IntegratorICVariant=InternalICs  ExternalResetVariant=Disabled  TRSumVariant=Passthrough  SumFdbkVariant=Disabled  SumVariant=Sum_PID  TsampFilterVariant=InternalTs  TsampNgainVariant=Passthrough  TsampIntegralVariant=Passthrough  ExternalSaturationOutDataTypeStr=Inherit: Same as second input
  Pitch_acts : Subsystem
  Pitch_meas : Selector  InputPortWidth=10  IndexOptions=Index vector (dialog)  Indices=[6]  OutputSizes=1
  Pitch_ref : Selector  InputPortWidth=4  IndexOptions=Index vector (dialog)  Indices=[3]  OutputSizes=1
  Pitch_sat : Saturate  UpperLimit=deg2rad(30)  LowerLimit=-deg2rad(30)
  Power : Math  Operator=pow
  Power1 : Math  Operator=pow
  Power2 : Math  Operator=pow
  Product : Product  Multiplication=Matrix(*)
  Product{1,3..5} (4 alike) : Product
  Product2 : Product  Multiplication=Matrix(*)
  R2D{,1..3} (4 alike) : simulink_extras/Transformations/Radians to Degrees
  Radians to Degrees{,2..4,6..12} (11 alike) : simulink_extras/Transformations/Radians to Degrees
  Roll_acts : Subsystem
  Roll_meas : Selector  InputPortWidth=10  IndexOptions=Index vector (dialog)  Indices=[5]  OutputSizes=1
  Roll_ref1 : Selector  InputPortWidth=4  IndexOptions=Index vector (dialog)  Indices=[3]  OutputSizes=1
  Roll_sat : Saturate  UpperLimit=deg2rad(30)  LowerLimit=-deg2rad(30)
  Saturation : Saturate  UpperLimit=deg2rad(45)  LowerLimit=-deg2rad(45)
  Scope : Scope  NumInputPorts=6
  Scope1 : Scope  NumInputPorts=4
  Selector1 : Selector  InputPortWidth=10  IndexOptions=Index vector (dialog)  Indices=[7 8]  OutputSizes=1
  Sin1 : Trigonometry
  Sqrt : Sqrt
  Step : Step  Time=3  SampleTime=0
  Step1 : Step  Time=5  SampleTime=0
  Step2 : Step  Time=6  SampleTime=0
  Step3 : Step  Time=8  SampleTime=0
  Step4 : Step  Time=3  SampleTime=0
  Step5 : Step  Time=6  SampleTime=0
  Subsystem : Subsystem
  Subsystem1 : Subsystem  Commented=on
  Sum{,2,5,7..9,13,16,18..20,22} (12 alike) : Sum  Inputs=++|
  Sum{1,3..4,6,10..12,14..15,17,21,23..24,26} (14 alike) : Sum  Inputs=|+-
  Sum25 : Sum  Inputs=|-+
  Sum27 : Sum  Inputs=|--+
  Terminator{2..7} (6 alike) : Terminator
  Thrust : Constant  Value=30
  Transfer Fcn : TransferFcn  Numerator=[100]  Denominator=[1 100]
  V_x_ref : Selector  InputPortWidth=4  IndexOptions=Index vector (dialog)  Indices=[2]  OutputSizes=1
  V_y_ref : Selector  InputPortWidth=4  IndexOptions=Index vector (dialog)  Indices=[2]  OutputSizes=1
  Vx_meas : Selector  InputPortWidth=10  IndexOptions=Index vector (dialog)  Indices=[3]  OutputSizes=1
  Vy_meas : Selector  InputPortWidth=10  IndexOptions=Index vector (dialog)  Indices=[4]  OutputSizes=1
  Wx_meas : Selector  InputPortWidth=10  IndexOptions=Index vector (dialog)  Indices=[8]  OutputSizes=1
  Wx_ref1 : Selector  InputPortWidth=4  IndexOptions=Index vector (dialog)  Indices=[4]  OutputSizes=1
  Wx_sat : Saturate  UpperLimit=deg2rad(300)  LowerLimit=-deg2rad(300)
  Wy_meas : Selector  InputPortWidth=10  IndexOptions=Index vector (dialog)  Indices=[9]  OutputSizes=1
  Wy_ref : Selector  InputPortWidth=4  IndexOptions=Index vector (dialog)  Indices=[4]  OutputSizes=1
  Wy_sat : Saturate  UpperLimit=deg2rad(300)  LowerLimit=-deg2rad(300)
  Wz_meas : Selector  InputPortWidth=10  IndexOptions=Index vector (dialog)  Indices=[10]  OutputSizes=1
  Wz_ref : Selector  InputPortWidth=2  IndexOptions=Index vector (dialog)  Indices=[2]  OutputSizes=1
  Wz_sat : Saturate  UpperLimit=deg2rad(120)  LowerLimit=-deg2rad(120)
  X_meas : Selector  InputPortWidth=10  IndexOptions=Index vector (dialog)  Indices=[1]  OutputSizes=1
  X_ref : Selector  InputPortWidth=4  IndexOptions=Index vector (dialog)  Indices=[1]  OutputSizes=1
  Y_meas : Selector  InputPortWidth=10  IndexOptions=Index vector (dialog)  Indices=[2]  OutputSizes=1
  Y_ref : Selector  InputPortWidth=4  IndexOptions=Index vector (dialog)  Indices=[1]  OutputSizes=1
  Yaw_acts : Subsystem
  xdot = Ax+Bu+G : Subsystem
  wires:
  Step1/1 -> Sum3/2
  Step/1 -> Sum3/1
  Constant/1 -> X_ref/1, Wy_ref/1, Pitch_ref/1, V_x_ref/1  "REF"
  V_x_ref/1 -> Sum7/2
  Sum3/1 -> GainImpulse/1  "V_x_impulse"
  Sum/1 -> Sum1/1  "Vx_set"
  Sum1/1 -> OuterLoop_Vx/1  "Err_Vx"
  Vx_meas/1 -> Sum1/2, [Vx_measured]
  OuterLoop_Vx/1 -> Gain_Pitch/1  "Pitch_desired"
  Gain_Pitch/1 -> Sum2/2
  Pitch_ref/1 -> Sum2/1
  Sum2/1 -> Pitch_sat/1  "Pitch_Set"
  Sum4/1 -> Gain_Rates/1
  Gain_Rates/1 -> MiddleLoop_Pitch/1  "Err_Pitch"
  Sum5/1 -> Wy_sat/1  "Wy_Set"
  MiddleLoop_Pitch/1 -> Sum5/2  "Wy_desired"
  Wy_ref/1 -> Sum5/1
  Gain_wy_err/1 -> InnerLoop_Wy/1, Errors/1  "err_Wy"
  Sum6/1 -> Gain_wy_err/1
  GainImpulse/1 -> Sum7/1, [Vel_ref], Integrator/1
  Pitch_meas/1 -> [Pitch_measured], Sum4/2
  Wy_meas/1 -> [Wy_measured], Sum6/2
  [Wy_measured] -> R2D/1  "Wy_meas"
  [Pitch_measured] -> Radians to Degrees3/1  "Pich_meas"
  [Vx_measured] -> Mux2/2  "Vx_meas"
  [My] -> Mux4/1  "My"
  R2D/1 -> Feedback Pitch/4  "Wy_meas"
  Radians to Degrees3/1 -> Feedback Pitch/3  "Pitch_meas"
  InnerLoop_Wy/1 -> Pitch_acts/2(My), [My]  "My"
  Demux/2 -> [Eps_Y]
  [Eps_Y] -> R2D1/1
  R2D1/1 -> Feedback Pitch/5  "Eps_meas"
  Mux5/1 -> xdot = Ax+Bu+G/2(u)  "u"
  xdot = Ax+Bu+G/2(ydot) -> Selector1/1
  Wy_sat/1 -> Sum6/1
  Pitch_sat/1 -> Sum4/1
  Sum7/1 -> Sum/1
  ExoLoop_Z/1 -> Gain_Vx/1  "Vx_des"
  X_ref/1 -> Sum8/2
  Integrator/1 -> Sum8/1, [X_Ref]
  Sum8/1 -> Sum10/1  "X_Set"
  Sum10/1 -> ExoLoop_Z/1  "X_err"
  X_meas/1 -> [X_meas], Sum10/2
  [Vel_ref] -> Mux2/1  "Vel_ref"
  Mux2/1 -> Feedback Pitch/2
  [X_meas] -> Mux3/2  "X_meas"
  [X_Ref] -> Mux3/1  "X_ref"
  Mux3/1 -> Feedback Pitch/1
  Gain_Vx/1 -> Sum/2
  [delta_y] -> Feedback Pitch/8  "delta_y"
  [Fx] -> Feedback Pitch/7  "Fx"
  Thrust/1 -> [Thrust], Pitch_acts/1(Thrust)
  Mux4/1 -> Feedback Pitch/6
  [My_sat] -> Mux4/2  "My_sat"
  [Thrust] -> Roll_acts/1(Thrust)
  Gain_Vy/1 -> Sum9/2
  Y_meas/1 -> Sum12/2, [Y_meas]
  Sum12/1 -> ExoLoop_Y/1  "Y_err"
  Sum19/1 -> Sum12/1  "Y_Set"
  Integrator1/1 -> [Y_Ref], Sum19/1
  Y_ref/1 -> Sum19/2
  ExoLoop_Y/1 -> Gain_Vy/1  "Vy_des"
  Sum18/1 -> Sum9/1
  Roll_sat/1 -> Sum15/1
  Wx_sat/1 -> Sum17/1
  InnerLoop_Wx/1 -> [Mx], Roll_acts/2(Mx)  "Mx"
  Wx_meas/1 -> Sum17/2, [Wx_measured]
  Roll_meas/1 -> Sum15/2, [Roll_measured]
  GainImpulse1/1 -> Integrator1/1, [Vel_y_ref], Sum18/1
  Sum17/1 -> Gain_wx_err/1
  Gain_wx_err/1 -> Errors_Wx/1, InnerLoop_Wx/1  "err_Wx"
  Wx_ref1/1 -> Sum16/1
  MiddleLoop_Roll/1 -> Sum16/2  "Wx_desired"
  Sum16/1 -> Wx_sat/1  "Wy_Set"
  Gain_RateWx/1 -> MiddleLoop_Roll/1  "Err_Roll"
  Sum15/1 -> Gain_RateWx/1
  Sum13/1 -> Roll_sat/1  "Roll_Set"
  Roll_ref1/1 -> Sum13/1
  Gain_Roll/1 -> Sum13/2
  OuterLoop_Vy/1 -> Gain_Roll/1  "Roll_desired"
  Vy_meas/1 -> [Vy_measured], Sum11/2
  Sum11/1 -> OuterLoop_Vy/1  "Err_Vy"
  Sum9/1 -> Sum11/1  "Vy_set"
  Sum14/1 -> GainImpulse1/1  "V_y_impulse"
  V_y_ref/1 -> Sum18/2
  Constant1/1 -> V_y_ref/1, Roll_ref1/1, Wx_ref1/1, Y_ref/1  "REF"
  Step2/1 -> Sum14/1
  Step3/1 -> Sum14/2
  [Mx_sat] -> Gain1/1
  [My_sat] -> Terminator4/1
  Demux/1 -> [Eps_X]
  Selector1/1 -> Demux/1
  Demux3/1 -> Gain2/1, Terminator5/1
  Gain1/1 -> Mux5/3
  Gain/1 -> Mux5/2
  [Mx_sat] -> Mux8/2  "Mx_sat"
  Mux8/1 -> Feedback Roll/6
  [Fy] -> Feedback Roll/7  "Fy"
  [delta_x] -> Feedback Roll/8  "delta_x"
  Mux7/1 -> Feedback Roll/1
  [Y_Ref] -> Mux7/1  "Y_ref"
  [Y_meas] -> Mux7/2  "Y_meas"
  Mux6/1 -> Feedback Roll/2
  [Vel_y_ref] -> Mux6/1  "Vel_y_ref"
  R2D3/1 -> Feedback Roll/5  "EpsX_meas"
  [Eps_X] -> R2D3/1
  Radians to Degrees2/1 -> Feedback Roll/3  "Roll_meas"
  R2D2/1 -> Feedback Roll/4  "Wx_meas"
  [Mx] -> Mux8/1  "Mx"
  [Vy_measured] -> Mux6/2  "Vy_meas"
  [Roll_measured] -> Radians to Degrees2/1  "Roll_meas"
  [Wx_measured] -> R2D2/1  "Wx_meas"
  Gain3/1 -> Mux5/4
  Gain2/1 -> Mux5/1
  Sum20/1 -> Sum21/1  "Heading_set"
  Wz_ref/1 -> Sum22/1  "Wz_ref"
  Step5/1 -> Sum23/2
  Gain_HdgRates/1 -> Errors1/1, Hdg_rate_Loop/1  "Err_Wz"
  Sum21/1 -> OuterLoop_Hdg/1  "Err_Hdg"
  Constant2/1 -> Wz_ref/1, Hdg_ref/1  "REF"
  Sum24/1 -> Gain_HdgRates/1
  Hdg_meas/1 -> Sum21/2, [Hdg_measured]
  GainImpulse2/1 -> [Heading_ref], Degrees to Radians/1
  OuterLoop_Hdg/1 -> Gain_Hdg/1  "Wy_desired"
  Sum22/1 -> Wz_sat/1  "Wy_Set"
  Wz_sat/1 -> [Wz_setpnt], Sum24/1
  Hdg_ref/1 -> Sum20/2
  GainMoment/1 -> [Mz], Yaw_acts/2(Mz)  "u"
  Hdg_rate_Loop/1 -> GainMoment/1  "Moment"
  xdot = Ax+Bu+G/1(y) -> Hdg_meas/1, Wz_meas/1, xdot = Ax+Bu+G/1(x), Wy_meas/1, X_meas/1, Vx_meas/1, Pitch_meas/1, Vy_meas/1, Y_meas/1, Roll_meas/1, Wx_meas/1
  Step4/1 -> Sum23/1
  Gain_Hdg/1 -> Sum22/2
  Sum23/1 -> GainImpulse2/1  "Hdg_impulse"
  Wz_meas/1 -> [Wz_measured], Transfer Fcn/1
  Degrees to Radians/1 -> Sum20/1
  [Thrust] -> Yaw_acts/1(Thrust)
  Gain4/1 -> Mux5/5
  [Mz_sat] -> Terminator2/1
  Yaw_acts/1(delta) -> [delta_yaw], [delta_psi]
  Pitch_acts/1(delta_theta) -> [delta_theta]
  Roll_acts/1(delta_phi) -> [delta_phi]
  [delta_phi] -> Mux9/1
  [delta_theta] -> Mux9/2
  [delta_psi] -> Mux9/3
  Mux9/1 -> Product/2
  [Heading_ref] -> Mux10/1  "Hdg_ref"
  [Hdg_measured] -> Radians to Degrees7/1  "Hdg_meas"
  Mux10/1 -> Scope/1
  [Wz_setpnt] -> Radians to Degrees/1  "Hdg_ref"
  [Wz_measured] -> Radians to Degrees4/1  "Hdg_meas"
  Mux11/1 -> Scope/2
  Radians to Degrees/1 -> Mux11/1  "Wz_setpoint"
  Radians to Degrees4/1 -> Mux11/2  "Wz_meas"
  Radians to Degrees7/1 -> Mux10/2  "Hdg_meas"
  [delta_yaw] -> Radians to Degrees8/1
  [delta_psi] -> Radians to Degrees9/1
  Radians to Degrees8/1 -> Scope/3  "delta_yaw"
  Radians to Degrees9/1 -> Scope/4  "delta_psi"
  Actuator Distribution/1(Servos) -> Product/1
  Subsystem/1(InvServos) -> Display/1, Product2/1
  Levers/1(Levers) -> Product1/2
  Product2/1 -> Product1/1
  Product1/1 -> Product5/2
  Product/1 -> Saturation/1, Display1/1
  Saturation/1 -> Gain6/1, [delta_sat]
  Demux1/1 -> Sum25/1
  Demux1/4 -> Sum26/2
  Demux1/3 -> Sum25/2
  Demux1/2 -> Sum26/1
  Sum25/1 -> Product3/2
  Sum26/1 -> Product4/2
  Product4/1 -> Power1/1, Mux12/1
  Product3/1 -> Power/1, Mux12/2
  Mux12/1 -> Display2/1, [Forces]
  [Mz] -> Mux13/1  "Mz"
  [Mz_sat] -> Mux13/2  "Mz_sat"
  Mux13/1 -> Scope/5
  [Moments] -> Demux4/1  "Mx,My,Mz"
  Transfer Fcn/1 -> Sum24/2
  [Moments] -> Demux2/1
  Demux2/3 -> Gain4/1
  Demux2/1 -> Terminator3/1
  Demux2/2 -> Gain3/1
  [delta_phi] -> Radians to Degrees6/1
  [delta_theta] -> Radians to Degrees10/1
  [Forces] -> Demux3/1
  Demux3/2 -> Gain/1, Terminator6/1
  Demux3/3 -> Terminator7/1
  Power/1 -> Sum27/1
  Power1/1 -> Sum27/2
  Sum27/1 -> Sqrt/1
  Constant5/1 -> Power/2, Power1/2, Power2/2
  Power2/1 -> Sum27/3
  [delta_psi] -> Radians to Degrees11/1
  [delta_sat] -> Radians to Degrees12/1
  Radians to Degrees6/1 -> Scope1/1  "d_phi"
  Radians to Degrees10/1 -> Scope1/2  "d_theta"
  Radians to Degrees11/1 -> Scope1/3  "d_psi"
  Radians to Degrees12/1 -> Scope1/4
  Demux4/3 -> Scope/6  "Mz_mix"
  Demux4/2 -> Mux4/3  "My_mix"
  Demux4/1 -> Mux8/3  "Mx_mix"
  [Thrust] -> Gain5/1, Power2/1
  Product5/1 -> [Moments]
  Gain6/1 -> Sin1/1
  Sin1/1 -> Demux1/1, Product2/2
  Gain5/1 -> Product5/1, Product4/1, Product3/1
  Sqrt/1 -> Mux12/3

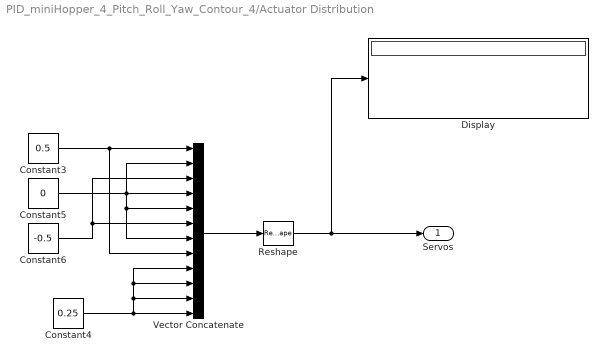
== system PID_miniHopper_4_Pitch_Roll_Yaw_Contour_4/Actuator Distribution ==
  Constant3 : Constant  Value=0.5
  Constant4 : Constant  Value=0.25
  Constant5 : Constant  Value=0
  Constant6 : Constant  Value=-0.5
  Display : Display
  Reshape : Reshape  OutputDimensionality=Customize  OutputDimensions=[4,3]
  Vector Concatenate : Concatenate  NumInputs=12
  Servos : Outport
  wires:
  Constant5/1 -> Vector Concatenate/7, Vector Concatenate/5, Vector Concatenate/4, Vector Concatenate/2
  Constant6/1 -> Vector Concatenate/6, Vector Concatenate/3
  Constant3/1 -> Vector Concatenate/8, Vector Concatenate/1
  Constant4/1 -> Vector Concatenate/9, Vector Concatenate/10, Vector Concatenate/11, Vector Concatenate/12
  Reshape/1 -> Servos/1, Display/1
  Vector Concatenate/1 -> Reshape/1

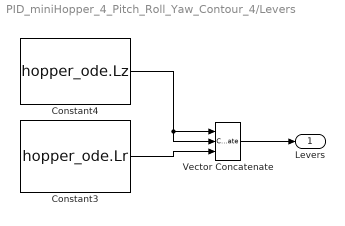
== system PID_miniHopper_4_Pitch_Roll_Yaw_Contour_4/Levers ==
  Constant3 : Constant  Value=hopper_ode.Lr
  Constant4 : Constant  Value=hopper_ode.Lz
  Vector Concatenate : Concatenate  NumInputs=3
  Levers : Outport
  wires:
  Constant4/1 -> Vector Concatenate/2, Vector Concatenate/1
  Constant3/1 -> Vector Concatenate/3
  Vector Concatenate/1 -> Levers/1

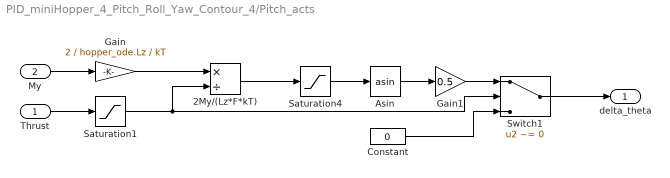
== system PID_miniHopper_4_Pitch_Roll_Yaw_Contour_4/Pitch_acts ==
  Thrust : Inport
  My : Inport  Port=2
  2My/(Lz*F*kT) : Product  Inputs=*/
  Asin : Trigonometry  Operator=asin
  Constant : Constant  Value=0
  Gain : Gain  Gain=2 / hopper_ode.Lz / kT
  Gain1 : Gain  Gain=0.5
  Saturation1 : Saturate  UpperLimit=25  LowerLimit=0
  Saturation4 : Saturate  UpperLimit=1  LowerLimit=-1
  Switch1 : Switch  Criteria=u2 ~= 0  SaturateOnIntegerOverflow=off  InputSameDT=off
  delta_theta : Outport
  wires:
  Gain/1 -> 2My/(Lz*F*kT)/1
  Switch1/1 -> delta_theta/1
  Constant/1 -> Switch1/3
  Thrust/1 -> Saturation1/1
  Saturation1/1 -> Switch1/2, 2My/(Lz*F*kT)/2
  Asin/1 -> Gain1/1
  Saturation4/1 -> Asin/1
  My/1 -> Gain/1
  2My/(Lz*F*kT)/1 -> Saturation4/1
  Gain1/1 -> Switch1/1

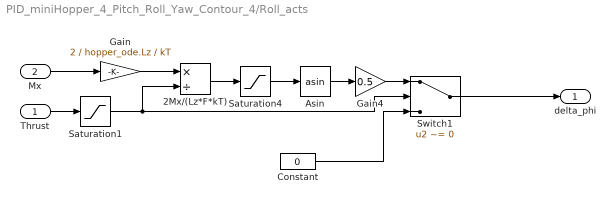
== system PID_miniHopper_4_Pitch_Roll_Yaw_Contour_4/Roll_acts ==
  Thrust : Inport
  Mx : Inport  Port=2
  2Mx/(Lz*F*kT) : Product  Inputs=*/
  Asin : Trigonometry  Operator=asin
  Constant : Constant  Value=0
  Gain : Gain  Gain=2 / hopper_ode.Lz / kT
  Gain4 : Gain  Gain=0.5
  Saturation1 : Saturate  UpperLimit=25  LowerLimit=0
  Saturation4 : Saturate  UpperLimit=1  LowerLimit=-1
  Switch1 : Switch  Criteria=u2 ~= 0  SaturateOnIntegerOverflow=off  InputSameDT=off
  delta_phi : Outport
  wires:
  Saturation4/1 -> Asin/1
  Asin/1 -> Gain4/1
  Saturation1/1 -> Switch1/2, 2Mx/(Lz*F*kT)/2
  Thrust/1 -> Saturation1/1
  Constant/1 -> Switch1/3
  Switch1/1 -> delta_phi/1
  2Mx/(Lz*F*kT)/1 -> Saturation4/1
  Gain/1 -> 2Mx/(Lz*F*kT)/1
  Mx/1 -> Gain/1
  Gain4/1 -> Switch1/1

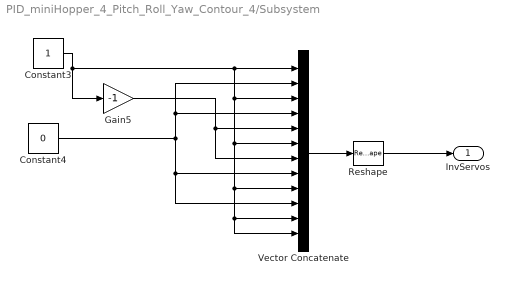
== system PID_miniHopper_4_Pitch_Roll_Yaw_Contour_4/Subsystem ==
  Constant3 : Constant
  Constant4 : Constant  Value=0
  Gain5 : Gain  Gain=-1
  Reshape : Reshape  OutputDimensionality=Customize  OutputDimensions=[3,4]
  Vector Concatenate : Concatenate  NumInputs=12
  InvServos : Outport
  wires:
  Constant3/1 -> Vector Concatenate/1, Vector Concatenate/12, Vector Concatenate/11, Vector Concatenate/9, Vector Concatenate/6, Vector Concatenate/3, Gain5/1
  Constant4/1 -> Vector Concatenate/2, Vector Concatenate/4, Vector Concatenate/10, Vector Concatenate/8
  Vector Concatenate/1 -> Reshape/1
  Gain5/1 -> Vector Concatenate/7, Vector Concatenate/5
  Reshape/1 -> InvServos/1

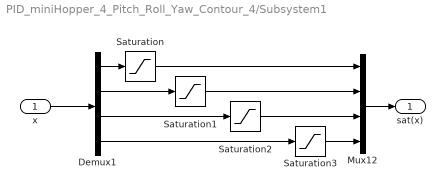
== system PID_miniHopper_4_Pitch_Roll_Yaw_Contour_4/Subsystem1 ==
  x : Inport
  Demux1 : Demux
  Mux12 : Mux
  Saturation{,1..3} (4 alike) : Saturate  UpperLimit=deg2rad(45)  LowerLimit=-deg2rad(45)
  sat(x) : Outport
  wires:
  Demux1/3 -> Saturation2/1
  Demux1/4 -> Saturation3/1
  Demux1/1 -> Saturation/1
  Demux1/2 -> Saturation1/1
  x/1 -> Demux1/1
  Mux12/1 -> sat(x)/1
  Saturation/1 -> Mux12/1
  Saturation1/1 -> Mux12/2
  Saturation2/1 -> Mux12/3
  Saturation3/1 -> Mux12/4

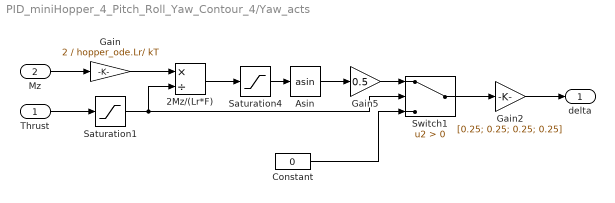
== system PID_miniHopper_4_Pitch_Roll_Yaw_Contour_4/Yaw_acts ==
  Thrust : Inport
  Mz : Inport  Port=2
  2Mz/(Lr*F) : Product  Inputs=*/
  Asin : Trigonometry  Operator=asin
  Constant : Constant  Value=0
  Gain : Gain  Gain=2 / hopper_ode.Lr/ kT
  Gain2 : Gain  Gain=[0.25; 0.25; 0.25; 0.25]
  Gain5 : Gain  Gain=0.5
  Saturation1 : Saturate  UpperLimit=25  LowerLimit=0
  Saturation4 : Saturate  UpperLimit=1  LowerLimit=-1
  Switch1 : Switch  Criteria=u2 > Threshold  SaturateOnIntegerOverflow=off  InputSameDT=off
  delta : Outport
  wires:
  Mz/1 -> Gain/1
  Gain/1 -> 2Mz/(Lr*F)/1
  2Mz/(Lr*F)/1 -> Saturation4/1
  Switch1/1 -> Gain2/1
  Constant/1 -> Switch1/3
  Thrust/1 -> Saturation1/1
  Gain2/1 -> delta/1
  Saturation1/1 -> Switch1/2, 2Mz/(Lr*F)/2
  Asin/1 -> Gain5/1
  Saturation4/1 -> Asin/1
  Gain5/1 -> Switch1/1
